simulink model "CM700A_HwTq3Meas"  (R2013b)
settings: Solver=FixedStepDiscrete  SolverMode=SingleTasking  StartTime=0.0  StopTime=1  FixedStep=0.002  RelTol=1e-3
values from neighbouring files (symbols this model uses):
  ELECGLBPRM_HWTQOFFS_HWNWTMTR_F32 = DataDict.Constant    [CM700A_HwTq3Meas_DataDict.m]
  ELECGLBPRM_HWTQSATNLOWRLIM_HWNWTMTR_F32 = DataDict.Constant    [CM700A_HwTq3Meas_DataDict.m]
  ELECGLBPRM_HWTQSATNUPPRLIM_HWNWTMTR_F32 = DataDict.Constant    [CM700A_HwTq3Meas_DataDict.m]
  ELECGLBPRM_HWTQSCA_ULS_F32 = DataDict.Constant    [CM700A_HwTq3Meas_DataDict.m]
  ELECGLBPRM_NOFLT_CNT_U08 = DataDict.Constant    [CM700A_HwTq3Meas_DataDict.m]
  ELECGLBPRM_OFFSTRIMNOTPRFM_CNT_U08 = DataDict.Constant    [CM700A_HwTq3Meas_DataDict.m]
  ELECGLBPRM_PRTCLFLT_CNT_U08 = DataDict.Constant    [CM700A_HwTq3Meas_DataDict.m]
  ELECGLBPRM_SNSRINTFLT_CNT_U08 = DataDict.Constant    [CM700A_HwTq3Meas_DataDict.m]
  GearIdn2 = DataDict.OpSignal    [CM700A_HwTq3Meas_DataDict.m]
  HwTq3MeasHwTq3PrtclFltFailStep = DataDict.Calibration    [CM700A_HwTq3Meas_DataDict.m]
  HwTq3MeasHwTq3PrtclFltPassStep = DataDict.Calibration    [CM700A_HwTq3Meas_DataDict.m]
undefined symbols (not defined in the file or in its folder): NtcNr1, NtcSts1, sigbuilder_block, SigQlfr1
libraries: simulink x22, NxtrNvM x3
(part 3 of 3)

== system CM700A_HwTq3Meas/HwTq3Meas/HwTq3MeasPer1/SlowSerlDataRead/SlowSerlRead0/SlowSerlRead1 ==
  SlowSerlMsgID : Inport
  SlowSerlMsgData : Inport  Port=2
  Action Port : ActionPort  ActionType=then
  CopyRight2 : Subsystem  Description=|  mask(Copyright Information){none=on}
      | Copyright info block.                                               
      |                                                                     
      | Place copyright information at the top of every subsystem in design.
      mask prompts: none "No parameters"
      mask help: Place copyright information at the top of every subsystem in design.
      mask Display:
      | NxtrConf = 'Nexteer Confidential';
      | 
      | sys = bdroot; %handle for the current model ("system")
      | first = get_param(sys,'Created');
      | first = first(end-3:end);  %year is last four digits
      | 
      | last = get_param(sys,'LastModifiedDate');
      | if isempty(last)
      |     last = datestr(now,'yyyy');
      | else
      |     last = last(end-3:end);
      | end
      | 
      | if strcmp(first,last)
      |     fprintf('%s -- Copyright %s Nexteer',NxtrConf,first)
      | else
      |     fprintf('%s -- %s%s- %s Nexteer',NxtrConf,char(169),first,last)
      | end
  If : If  IfExpression=(u1==2)  ShowElse=off
  SlowSerlRead2 : Subsystem  TreatAsAtomicUnit=on
  wires:
  If/1 -> SlowSerlRead2/Action
  SlowSerlMsgID/1 -> If/1
  SlowSerlMsgData/1 -> SlowSerlRead2/1(SlowSerlMsgData)

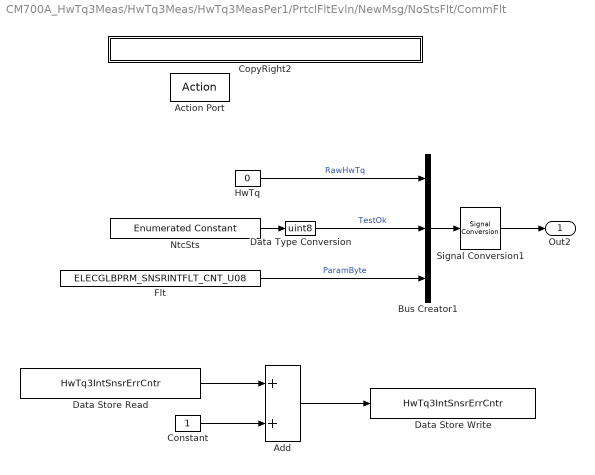
== system CM700A_HwTq3Meas/HwTq3Meas/HwTq3MeasPer1/PrtclFltEvln/NewMsg/NoStsFlt/CommFlt ==
  Action Port : ActionPort  ActionType=else
  Add : Sum
  Bus Creator1 : BusCreator  Inputs=3
  Constant : Constant  OutDataTypeStr=uint8
  CopyRight2 : Subsystem  Description=|  mask(Copyright Information){none=on}
      | Copyright info block.                                               
      |                                                                     
      | Place copyright information at the top of every subsystem in design.
      mask prompts: none "No parameters"
      mask help: Place copyright information at the top of every subsystem in design.
      mask Display:
      | NxtrConf = 'Nexteer Confidential';
      | 
      | sys = bdroot; %handle for the current model ("system")
      | first = get_param(sys,'Created');
      | first = first(end-3:end);  %year is last four digits
      | 
      | last = get_param(sys,'LastModifiedDate');
      | if isempty(last)
      |     last = datestr(now,'yyyy');
      | else
      |     last = last(end-3:end);
      | end
      | 
      | if strcmp(first,last)
      |     fprintf('%s -- Copyright %s Nexteer',NxtrConf,first)
      | else
      |     fprintf('%s -- %s%s- %s Nexteer',NxtrConf,char(169),first,last)
      | end
  Data Store Read : DataStoreRead  DataStoreName=HwTq3IntSnsrErrCntr
  Data Store Write : DataStoreWrite  DataStoreName=HwTq3IntSnsrErrCntr
  Data Type Conversion : DataTypeConversion  OutDataTypeStr=uint8
  Flt : Constant  Value=ELECGLBPRM_SNSRINTFLT_CNT_U08  OutDataTypeStr=uint8
  HwTq : Constant  Value=0  OutDataTypeStr=uint32
  NtcSts : simulink/Sources/Enumerated Constant  OutDataTypeStr=Enum: NtcSts1  Value=NtcSts1.NTCSTS_PREFAILD  SampleTime=inf
  Signal Conversion1 : SignalConversion
  Out2 : Outport
  wires:
  Flt/1 -> Bus Creator1/3  "ParamByte"
  NtcSts/1 -> Data Type Conversion/1
  HwTq/1 -> Bus Creator1/1  "RawHwTq"
  Bus Creator1/1 -> Signal Conversion1/1
  Signal Conversion1/1 -> Out2/1
  Data Type Conversion/1 -> Bus Creator1/2  "TestOk"
  Data Store Read/1 -> Add/1
  Constant/1 -> Add/2
  Add/1 -> Data Store Write/1

== system CM700A_HwTq3Meas/HwTq3Meas/HwTq3MeasPer1/PrtclFltEvln/NewMsg/NoStsFlt/CopyRight2 ==

== system CM700A_HwTq3Meas/HwTq3Meas/HwTq3MeasPer1/PrtclFltEvln/NewMsg/NoStsFlt/TestPass ==
  RegInpRSENT5ND : Inport
  Action Port : ActionPort  ActionType=then
  Bus Creator : BusCreator  Inputs=3
  CopyRight2 : Subsystem  Description=|  mask(Copyright Information){none=on}
      | Copyright info block.                                               
      |                                                                     
      | Place copyright information at the top of every subsystem in design.
      mask prompts: none "No parameters"
      mask help: Place copyright information at the top of every subsystem in design.
      mask Display:
      | NxtrConf = 'Nexteer Confidential';
      | 
      | sys = bdroot; %handle for the current model ("system")
      | first = get_param(sys,'Created');
      | first = first(end-3:end);  %year is last four digits
      | 
      | last = get_param(sys,'LastModifiedDate');
      | if isempty(last)
      |     last = datestr(now,'yyyy');
      | else
      |     last = last(end-3:end);
      | end
      | 
      | if strcmp(first,last)
      |     fprintf('%s -- Copyright %s Nexteer',NxtrConf,first)
      | else
      |     fprintf('%s -- %s%s- %s Nexteer',NxtrConf,char(169),first,last)
      | end
  Data Type Conversion : DataTypeConversion  OutDataTypeStr=uint8
  Data Type Conversion1 : DataTypeConversion  OutDataTypeStr=uint32
  NoFlt : Constant  RequirementInfo={} %GIDa_e64df96d_f0ef_4edd_b9a4_9c46566b9362  Value=ELECGLBPRM_NOFLT_CNT_U08  OutDataTypeStr=uint8
  NtcSts1 : simulink/Sources/Enumerated Constant  OutDataTypeStr=Enum: NtcSts1  Value=NtcSts1.NTCSTS_PREPASSD  SampleTime=inf
  Signal Conversion : SignalConversion
  Out1 : Outport
  wires:
  NtcSts1/1 -> Data Type Conversion/1
  Data Type Conversion/1 -> Bus Creator/2  "TestOk"
  NoFlt/1 -> Bus Creator/3  "ParamByte"
  RegInpRSENT5ND/1 -> Data Type Conversion1/1  "RawHwTq"
  Bus Creator/1 -> Signal Conversion/1
  Data Type Conversion1/1 -> Bus Creator/1  "RawHwTq"
  Signal Conversion/1 -> Out1/1

== system CM700A_HwTq3Meas/HwTq3Meas/HwTq3MeasPer1/PrtclFltEvln/NewMsg/StsFlt/CopyRight2 ==

== system CM700A_HwTq3Meas/HwTq3Meas/HwTq3MeasPer1/SlowSerlDataRead/SlowSerlRead0/SlowSerlRead1/CopyRight2 ==

== system CM700A_HwTq3Meas/HwTq3Meas/HwTq3MeasPer1/SlowSerlDataRead/SlowSerlRead0/SlowSerlRead1/SlowSerlRead2 ==
  SlowSerlMsgData : Inport
  Action Port : ActionPort  ActionType=then
  Constant : Constant  Value=true  OutDataTypeStr=boolean
      settings: AttributesFormatString=%<OutDataTypeStr>
  CopyRight2 : Subsystem  Description=|  mask(Copyright Information){none=on}
      | Copyright info block.                                               
      |                                                                     
      | Place copyright information at the top of every subsystem in design.
      mask prompts: none "No parameters"
      mask help: Place copyright information at the top of every subsystem in design.
      mask Display:
      | NxtrConf = 'Nexteer Confidential';
      | 
      | sys = bdroot; %handle for the current model ("system")
      | first = get_param(sys,'Created');
      | first = first(end-3:end);  %year is last four digits
      | 
      | last = get_param(sys,'LastModifiedDate');
      | if isempty(last)
      |     last = datestr(now,'yyyy');
      | else
      |     last = last(end-3:end);
      | end
      | 
      | if strcmp(first,last)
      |     fprintf('%s -- Copyright %s Nexteer',NxtrConf,first)
      | else
      |     fprintf('%s -- %s%s- %s Nexteer',NxtrConf,char(169),first,last)
      | end
  Data1 : DataStoreWrite  DataStoreName=GearIdn2Avl
  Data2 : DataStoreWrite  DataStoreName=GearIdn2Data
  wires:
  Constant/1 -> Data1/1
  SlowSerlMsgData/1 -> Data2/1

== system CM700A_HwTq3Meas/HwTq3Meas/HwTq3MeasPer1/PrtclFltEvln/NewMsg/NoStsFlt/CommFlt/CopyRight2 ==

== system CM700A_HwTq3Meas/HwTq3Meas/HwTq3MeasPer1/PrtclFltEvln/NewMsg/NoStsFlt/TestPass/CopyRight2 ==

== system CM700A_HwTq3Meas/HwTq3Meas/HwTq3MeasPer1/SlowSerlDataRead/SlowSerlRead0/SlowSerlRead1/SlowSerlRead2/CopyRight2 ==

== stateflow chart CM700A_HwTq3Meas/HwTq3Meas/HwTq3MeasPer2/SetNtcSts/ISO Fault Debounce Design ==
  settings: stateMachineType=MEALY_MACHINE
  note: NTCSTS_PASSD           (0)
      | NTCSTS_FAILD             (1)
      | NTCSTS_PREPASSD   (2)
      | NTCSTS_PREFAILD     (3)
      |
      | SIGQLFR_NORES        (0)
      | SIGQLFR_PASSD         (1)
      | SIGQLFR_FAILD           (2)
  note: Pass Loop
  note: Fail Loop
  note: 
  (default) -> (junction 89)
  (junction 89) -> (junction 95) [order 1] : [NtcSts ==3]
  (junction 89) -> (junction 93) [order 2] : [NtcSts ==2]
  (junction 89) -> (junction 141) [order 3] : [NtcSts ==1]
      | { ErrAcc = 32767;
      | Qualifier =2;
      |  }
  (junction 89) -> (junction 141) [order 4] : [NtcSts ==0]
      | { ErrAcc = -32768;
      | Qualifier=1;
      | }
  (junction 95) -> (junction 103) [order 2]
  (junction 95) -> (junction 111) [order 1] : [ErrAcc <=0]
      | {ErrAcc = DebStep;}
  (junction 93) -> (junction 123) [order 2] : {
      | ErrAcc = ErrAcc - DebStep;
      | }
  (junction 93) -> (junction 123) [order 1] : [(ErrAcc - DebStep) <= -32768]
      | { ErrAcc = -32768;
      | Qualifier=1;
      | }
  (junction 103) -> (junction 111) [order 1] : [(ErrAcc + DebStep) <32767]
      | {ErrAcc = ErrAcc + DebStep;}
  (junction 103) -> (junction 111) [order 2] : {ErrAcc = 32767;
      | Qualifier =2;}
  (junction 123) -> (junction 141)
  (junction 111) -> (junction 141)
  (junction 141) -> (junction 159) [order 2] : {ErrAcc = 0;
      | Qualifier =0;
      | }
  (junction 141) -> (junction 159) [order 1] : [SvcClr ==0]
  data: NtcSts input uint8; Qualifier output uint8; DebStep input uint16; ErrAcc local single; SvcClr input

== stateflow chart CM700A_HwTq3Meas/HwTq3Meas/HwTq3MeasPer1/SetNtcSts/ISO Fault Debounce Design ==
  settings: stateMachineType=MEALY_MACHINE
  note: NTCSTS_PASSD           (0)
      | NTCSTS_FAILD             (1)
      | NTCSTS_PREPASSD   (2)
      | NTCSTS_PREFAILD     (3)
      |
      | SIGQLFR_NORES        (0)
      | SIGQLFR_PASSD         (1)
      | SIGQLFR_FAILD           (2)
  note: Pass Loop
  note: Fail Loop
  note: 
  (default) -> (junction 89)
  (junction 89) -> (junction 95) [order 1] : [NtcSts ==3]
  (junction 89) -> (junction 93) [order 2] : [NtcSts ==2]
  (junction 89) -> (junction 141) [order 3] : [NtcSts ==1]
      | { ErrAcc = 32767;
      | Qualifier =2;
      |  }
  (junction 89) -> (junction 141) [order 4] : [NtcSts ==0]
      | { ErrAcc = -32768;
      | Qualifier=1;
      | }
  (junction 95) -> (junction 103) [order 2]
  (junction 95) -> (junction 111) [order 1] : [ErrAcc <=0]
      | {ErrAcc = DebStep;}
  (junction 93) -> (junction 123) [order 2] : {
      | ErrAcc = ErrAcc - DebStep;
      | }
  (junction 93) -> (junction 123) [order 1] : [(ErrAcc - DebStep) <= -32768]
      | { ErrAcc = -32768;
      | Qualifier=1;
      | }
  (junction 103) -> (junction 111) [order 1] : [(ErrAcc + DebStep) <32767]
      | {ErrAcc = ErrAcc + DebStep;}
  (junction 103) -> (junction 111) [order 2] : {ErrAcc = 32767;
      | Qualifier =2;}
  (junction 123) -> (junction 141)
  (junction 111) -> (junction 141)
  (junction 141) -> (junction 159) [order 2] : {ErrAcc = 0;
      | Qualifier =0;
      | }
  (junction 141) -> (junction 159) [order 1] : [SvcClr ==0]
  data: NtcSts input uint8; Qualifier output uint8; DebStep input uint16; ErrAcc local int16; SvcClr input

== stateflow chart CM700A_HwTq3Meas/HwTq3Meas/HwTq3MeasPer1/RollCnt1 ==
  settings: stateMachineType=MEALY_MACHINE
  (default) -> (junction 89) : {HwTq3RollgCntr = HwTq3PrevRollgCntr;}
  (junction 89) -> (junction 169) [order 1] : [ (TestOk ==2) ]
  (junction 89) -> (junction 93) [order 2]
  (junction 169) -> (junction 93) [order 2] : {HwTq3RollgCntr = 0;}
  (junction 169) -> (junction 93) [order 1] : [(HwTq3RollgCntr+1) <= 255]
      | {HwTq3RollgCntr = HwTq3RollgCntr + 1;}
  (junction 93) -> (junction 188)
  data: TestOk input uint8; HwTq3PrevRollgCntr input; HwTq3RollgCntr output uint8
